simulink model "CF012A_GmStrtStop"  (R2013b)
settings: Solver=FixedStepDiscrete  SolverMode=SingleTasking  StartTime=0.0  StopTime=1  FixedStep=0.002  RelTol=1e-3
values from neighbouring files (symbols this model uses):
  CNV100MICROSECTOMILLISEC_MILLISECPERCNT_F32 = DataDict.Constant    [CF012A_GmStrtStop_DataDict.m]
  DISMOD_CNT_U08 = DataDict.Constant    [CF012A_GmStrtStop_DataDict.m]
  DISMODRATE_ULSPERSEC_F32 = DataDict.Constant    [CF012A_GmStrtStop_DataDict.m]
  FLTMOD_CNT_U08 = DataDict.Constant    [CF012A_GmStrtStop_DataDict.m]
  GmStrtStopEna = DataDict.Calibration    [CF012A_GmStrtStop_DataDict.m]
  GmStrtStopFltRateLim = DataDict.Calibration    [CF012A_GmStrtStop_DataDict.m]
  GmStrtStopMod1ToStopRateLim = DataDict.Calibration    [CF012A_GmStrtStop_DataDict.m]
  GmStrtStopNormRateLim = DataDict.Calibration    [CF012A_GmStrtStop_DataDict.m]
  GmStrtStopNormToMod1RateLim = DataDict.Calibration    [CF012A_GmStrtStop_DataDict.m]
  GmStrtStopStopAndMod2RateLim = DataDict.Calibration    [CF012A_GmStrtStop_DataDict.m]
  GmStrtStopStopMod1Tmr = DataDict.Calibration    [CF012A_GmStrtStop_DataDict.m]
  GmStrtStopStopMod2Tmr = DataDict.Calibration    [CF012A_GmStrtStop_DataDict.m]
  MOD1_CNT_U08 = DataDict.Constant    [CF012A_GmStrtStop_DataDict.m]
  MOD2_CNT_U08 = DataDict.Constant    [CF012A_GmStrtStop_DataDict.m]
  NORMMOD_CNT_U08 = DataDict.Constant    [CF012A_GmStrtStop_DataDict.m]
  STOPMOD_CNT_U08 = DataDict.Constant    [CF012A_GmStrtStop_DataDict.m]
  STRTSTOPRATEHILIM_ULSPERSEC_F32 = DataDict.Constant    [CF012A_GmStrtStop_DataDict.m]
  STRTSTOPRATELOWRLIM_ULSPERSEC_F32 = DataDict.Constant    [CF012A_GmStrtStop_DataDict.m]
  STRTSTOPSCAHILIM_ULS_F32 = DataDict.Constant    [CF012A_GmStrtStop_DataDict.m]
  STRTSTOPSCALOWRLIM_ULS_F32 = DataDict.Constant    [CF012A_GmStrtStop_DataDict.m]
undefined symbols (not defined in the file or in its folder): u2, u3, u4, u5
libraries: FixdToFloat x2, NxtrLim x2, simulink x2
(part 2 of 4)

== system CF012A_GmStrtStop/GmStrtStop/GmStrtStopPer1/DtrmnPrevActSt ==
  note: /*** Set PrevStrtStopSt read/write priority to fix bug, no software change required ***/
  StrtStopSt : Inport  RequirementInfo="{'linktype_rmi_doors' '0000c6e0 (/GM T1XX/SubSystem Specifications/Customer Functions/CF012 12V Start Stop)' '#186' 'true' 'REQ:  186' '' ; 'linktype_rmi_doors' '0000c6e0 (/GM T1XX/SubSystem Specifications/Customer Functions/CF012 12V Start Stop)' '#148' 'true' 'REQ:  148' '' ; 'linktype_rmi_doors' '0000c6e0 (/GM T1XX/SubSystem Specifications/Customer Functions/CF012 12V Start Stop)' '#148' 'true' 'REQ:  148' '' ; 'linktype_rmi_doors' '0000c6e0 (/GM T1XX/SubSystem Specifications/Customer Functions/CF012 12V Start Stop)' '#148' 'true' 'REQ:  148' '' ; 'linktype_rmi_doors' '0000c6e0 (/GM T1XX/SubSystem Specifications/Customer Functions/CF012 12V Start Stop)' '#148' 'true' 'REQ:  148' '' ; 'linktype_rmi_doors' '0000c6e0 (/GM T1XX/SubSystem Specifications/Customer Functions/CF012 12V Start Stop)' '#148' 'true' 'REQ:  148' '' ; 'linktype_rmi_doors' '0000c6e0 (/GM T1XX/SubSystem Specifications/Customer Functions/CF012 12V Start Stop)' '#148' 'true' 'REQ:  148' '' ; 'linktype_rmi_doors' '0000c6e0 (/GM T1XX/SubSystem Specifications/Customer Functions/CF012 12V Start Stop)' '#148' 'true' 'REQ:  148' '' } %GIDa_e4f48af0_6723_4855_972c_b2aebfcfadbe"
  CopyRight2 : Subsystem  Description=|  mask(Copyright Information){none=on}
      | Copyright info block.                                               
      |                                                                     
      | Place copyright information at the top of every subsystem in design.
      mask prompts: none "No parameters"
      mask help: Place copyright information at the top of every subsystem in design.
      mask Display:
      | NxtrConf = 'Nexteer Confidential';
      | 
      | sys = bdroot; %handle for the current model ("system")
      | first = get_param(sys,'Created');
      | if(isempty(first))
      |     first = datestr(now,'yyyy');
      | else
      |     first = first(end-3:end);  %year is last four digits
      | end
      | 
      | last = get_param(sys,'LastModifiedDate');
      | if isempty(last)
      |     last = datestr(now,'yyyy');
      | else
      |     last = last(end-3:end);
      | end
      | 
      | if strcmp(first,last)
      |     fprintf('%s -- Copyright %s Nexteer',NxtrConf,first)
      | else
      |     fprintf('%s -- %s%s- %s Nexteer',NxtrConf,char(169),first,last)
      | end
  Data Store Read : DataStoreRead  RequirementInfo="{'linktype_rmi_doors' '0000c6e0 (/GM T1XX/SubSystem Specifications/Customer Functions/CF012 12V Start Stop)' '#186' 'true' 'REQ:  186' '' ; 'linktype_rmi_doors' '0000c6e0 (/GM T1XX/SubSystem Specifications/Customer Functions/CF012 12V Start Stop)' '#148' 'true' 'REQ:  148' '' ; 'linktype_rmi_doors' '0000c6e0 (/GM T1XX/SubSystem Specifications/Customer Functions/CF012 12V Start Stop)' '#148' 'true' 'REQ:  148' '' ; 'linktype_rmi_doors' '0000c6e0 (/GM T1XX/SubSystem Specifications/Customer Functions/CF012 12V Start Stop)' '#148' 'true' 'REQ:  148' '' ; 'linktype_rmi_doors' '0000c6e0 (/GM T1XX/SubSystem Specifications/Customer Functions/CF012 12V Start Stop)' '#148' 'true' 'REQ:  148' '' ; 'linktype_rmi_doors' '0000c6e0 (/GM T1XX/SubSystem Specifications/Customer Functions/CF012 12V Start Stop)' '#148' 'true' 'REQ:  148' '' ; 'linktype_rmi_doors' '0000c6e0 (/GM T1XX/SubSystem Specifications/Customer Functions/CF012 12V Start Stop)' '#148' 'true' 'REQ:  148' '' ; 'linktype_rmi_doors' '0000c6e0 (/GM T1XX/SubSystem Specifications/Customer Functions/CF012 12V Start Stop)' '#148' 'true' 'REQ:  148' '' } %GIDa_4112967c_5abe_441b_ba9c_e70bf3192b6c"  Priority=0  DataStoreName=PrevStrtStopSt
      settings: AttributesFormatString=%<Priority>
  Data Store Write : DataStoreWrite  RequirementInfo="{'linktype_rmi_doors' '0000c6e0 (/GM T1XX/SubSystem Specifications/Customer Functions/CF012 12V Start Stop)' '#186' 'true' 'REQ:  186' '' ; 'linktype_rmi_doors' '0000c6e0 (/GM T1XX/SubSystem Specifications/Customer Functions/CF012 12V Start Stop)' '#148' 'true' 'REQ:  148' '' ; 'linktype_rmi_doors' '0000c6e0 (/GM T1XX/SubSystem Specifications/Customer Functions/CF012 12V Start Stop)' '#148' 'true' 'REQ:  148' '' ; 'linktype_rmi_doors' '0000c6e0 (/GM T1XX/SubSystem Specifications/Customer Functions/CF012 12V Start Stop)' '#148' 'true' 'REQ:  148' '' ; 'linktype_rmi_doors' '0000c6e0 (/GM T1XX/SubSystem Specifications/Customer Functions/CF012 12V Start Stop)' '#148' 'true' 'REQ:  148' '' ; 'linktype_rmi_doors' '0000c6e0 (/GM T1XX/SubSystem Specifications/Customer Functions/CF012 12V Start Stop)' '#148' 'true' 'REQ:  148' '' ; 'linktype_rmi_doors' '0000c6e0 (/GM T1XX/SubSystem Specifications/Customer Functions/CF012 12V Start Stop)' '#148' 'true' 'REQ:  148' '' ; 'linktype_rmi_doors' '0000c6e0 (/GM T1XX/SubSystem Specifications/Customer Functions/CF012 12V Start Stop)' '#148' 'true' 'REQ:  148' '' } %GIDa_cb98726f_60b3_46df_96ca_b94222df7bed"  Priority=1  DataStoreName=PrevStrtStopSt
      settings: AttributesFormatString=%<Priority>
  Data Store Write1 : DataStoreWrite  RequirementInfo="{'linktype_rmi_doors' '0000c6e0 (/GM T1XX/SubSystem Specifications/Customer Functions/CF012 12V Start Stop)' '#186' 'true' 'REQ:  186' '' ; 'linktype_rmi_doors' '0000c6e0 (/GM T1XX/SubSystem Specifications/Customer Functions/CF012 12V Start Stop)' '#148' 'true' 'REQ:  148' '' ; 'linktype_rmi_doors' '0000c6e0 (/GM T1XX/SubSystem Specifications/Customer Functions/CF012 12V Start Stop)' '#148' 'true' 'REQ:  148' '' ; 'linktype_rmi_doors' '0000c6e0 (/GM T1XX/SubSystem Specifications/Customer Functions/CF012 12V Start Stop)' '#148' 'true' 'REQ:  148' '' ; 'linktype_rmi_doors' '0000c6e0 (/GM T1XX/SubSystem Specifications/Customer Functions/CF012 12V Start Stop)' '#148' 'true' 'REQ:  148' '' ; 'linktype_rmi_doors' '0000c6e0 (/GM T1XX/SubSystem Specifications/Customer Functions/CF012 12V Start Stop)' '#148' 'true' 'REQ:  148' '' ; 'linktype_rmi_doors' '0000c6e0 (/GM T1XX/SubSystem Specifications/Customer Functions/CF012 12V Start Stop)' '#148' 'true' 'REQ:  148' '' ; 'linktype_rmi_doors' '0000c6e0 (/GM T1XX/SubSystem Specifications/Customer Functions/CF012 12V Start Stop)' '#148' 'true' 'REQ:  148' '' } %GIDa_3c095796_580b_4ffd_824f_51ea0e0332a4"  DataStoreName=PrevActSt
  Merge : Merge  RequirementInfo="{'linktype_rmi_doors' '0000c6e0 (/GM T1XX/SubSystem Specifications/Customer Functions/CF012 12V Start Stop)' '#186' 'true' 'REQ:  186' '' ; 'linktype_rmi_doors' '0000c6e0 (/GM T1XX/SubSystem Specifications/Customer Functions/CF012 12V Start Stop)' '#148' 'true' 'REQ:  148' '' ; 'linktype_rmi_doors' '0000c6e0 (/GM T1XX/SubSystem Specifications/Customer Functions/CF012 12V Start Stop)' '#148' 'true' 'REQ:  148' '' ; 'linktype_rmi_doors' '0000c6e0 (/GM T1XX/SubSystem Specifications/Customer Functions/CF012 12V Start Stop)' '#148' 'true' 'REQ:  148' '' ; 'linktype_rmi_doors' '0000c6e0 (/GM T1XX/SubSystem Specifications/Customer Functions/CF012 12V Start Stop)' '#148' 'true' 'REQ:  148' '' ; 'linktype_rmi_doors' '0000c6e0 (/GM T1XX/SubSystem Specifications/Customer Functions/CF012 12V Start Stop)' '#148' 'true' 'REQ:  148' '' ; 'linktype_rmi_doors' '0000c6e0 (/GM T1XX/SubSystem Specifications/Customer Functions/CF012 12V Start Stop)' '#148' 'true' 'REQ:  148' '' ; 'linktype_rmi_doors' '0000c6e0 (/GM T1XX/SubSystem Specifications/Customer Functions/CF012 12V Start Stop)' '#148' 'true' 'REQ:  148' '' } %GIDa_01ea55aa_64ba_4614_8fef_670c876545a6"
  PassLastSt : Subsystem  RequirementInfo="{'linktype_rmi_doors' '0000c6e0 (/GM T1XX/SubSystem Specifications/Customer Functions/CF012 12V Start Stop)' '#186' 'true' 'REQ:  186' '' ; 'linktype_rmi_doors' '0000c6e0 (/GM T1XX/SubSystem Specifications/Customer Functions/CF012 12V Start Stop)' '#148' 'true' 'REQ:  148' '' ; 'linktype_rmi_doors' '0000c6e0 (/GM T1XX/SubSystem Specifications/Customer Functions/CF012 12V Start Stop)' '#148' 'true' 'REQ:  148' '' ; 'linktype_rmi_doors' '0000c6e0 (/GM T1XX/SubSystem Specifications/Customer Functions/CF012 12V Start Stop)' '#148' 'true' 'REQ:  148' '' ; 'linktype_rmi_doors' '0000c6e0 (/GM T1XX/SubSystem Specifications/Customer Functions/CF012 12V Start Stop)' '#148' 'true' 'REQ:  148' '' ; 'linktype_rmi_doors' '0000c6e0 (/GM T1XX/SubSystem Specifications/Customer Functions/CF012 12V Start Stop)' '#148' 'true' 'REQ:  148' '' ; 'linktype_rmi_doors' '0000c6e0 (/GM T1XX/SubSystem Specifications/Customer Functions/CF012 12V Start Stop)' '#148' 'true' 'REQ:  148' '' ; 'linktype_rmi_doors' '0000c6e0 (/GM T1XX/SubSystem Specifications/Customer Functions/CF012 12V Start Stop)' '#148' 'true' 'REQ:  148' '' } %GIDa_88907860_9b17_4b86_96c1_9ce7d81e5492"  TreatAsAtomicUnit=on
  PassPrevLoopRes : Subsystem  RequirementInfo="{'linktype_rmi_doors' '0000c6e0 (/GM T1XX/SubSystem Specifications/Customer Functions/CF012 12V Start Stop)' '#186' 'true' 'REQ:  186' '' ; 'linktype_rmi_doors' '0000c6e0 (/GM T1XX/SubSystem Specifications/Customer Functions/CF012 12V Start Stop)' '#148' 'true' 'REQ:  148' '' ; 'linktype_rmi_doors' '0000c6e0 (/GM T1XX/SubSystem Specifications/Customer Functions/CF012 12V Start Stop)' '#148' 'true' 'REQ:  148' '' ; 'linktype_rmi_doors' '0000c6e0 (/GM T1XX/SubSystem Specifications/Customer Functions/CF012 12V Start Stop)' '#148' 'true' 'REQ:  148' '' ; 'linktype_rmi_doors' '0000c6e0 (/GM T1XX/SubSystem Specifications/Customer Functions/CF012 12V Start Stop)' '#148' 'true' 'REQ:  148' '' ; 'linktype_rmi_doors' '0000c6e0 (/GM T1XX/SubSystem Specifications/Customer Functions/CF012 12V Start Stop)' '#148' 'true' 'REQ:  148' '' ; 'linktype_rmi_doors' '0000c6e0 (/GM T1XX/SubSystem Specifications/Customer Functions/CF012 12V Start Stop)' '#148' 'true' 'REQ:  148' '' ; 'linktype_rmi_doors' '0000c6e0 (/GM T1XX/SubSystem Specifications/Customer Functions/CF012 12V Start Stop)' '#148' 'true' 'REQ:  148' '' } %GIDa_c43dcfaf_7e1c_468a_acca_d131cc0d12a7"  TreatAsAtomicUnit=on
  Relational Operator : RelationalOperator  RequirementInfo="{'linktype_rmi_doors' '0000c6e0 (/GM T1XX/SubSystem Specifications/Customer Functions/CF012 12V Start Stop)' '#186' 'true' 'REQ:  186' '' ; 'linktype_rmi_doors' '0000c6e0 (/GM T1XX/SubSystem Specifications/Customer Functions/CF012 12V Start Stop)' '#148' 'true' 'REQ:  148' '' ; 'linktype_rmi_doors' '0000c6e0 (/GM T1XX/SubSystem Specifications/Customer Functions/CF012 12V Start Stop)' '#148' 'true' 'REQ:  148' '' ; 'linktype_rmi_doors' '0000c6e0 (/GM T1XX/SubSystem Specifications/Customer Functions/CF012 12V Start Stop)' '#148' 'true' 'REQ:  148' '' ; 'linktype_rmi_doors' '0000c6e0 (/GM T1XX/SubSystem Specifications/Customer Functions/CF012 12V Start Stop)' '#148' 'true' 'REQ:  148' '' ; 'linktype_rmi_doors' '0000c6e0 (/GM T1XX/SubSystem Specifications/Customer Functions/CF012 12V Start Stop)' '#148' 'true' 'REQ:  148' '' ; 'linktype_rmi_doors' '0000c6e0 (/GM T1XX/SubSystem Specifications/Customer Functions/CF012 12V Start Stop)' '#148' 'true' 'REQ:  148' '' ; 'linktype_rmi_doors' '0000c6e0 (/GM T1XX/SubSystem Specifications/Customer Functions/CF012 12V Start Stop)' '#148' 'true' 'REQ:  148' '' } %GIDa_d7497edc_1bfd_4ac3_af9a_a8a8c06f0d57"  Operator=~=  OutDataTypeStr=boolean
  StrtStopSt_IF : If  RequirementInfo="{'linktype_rmi_doors' '0000c6e0 (/GM T1XX/SubSystem Specifications/Customer Functions/CF012 12V Start Stop)' '#186' 'true' 'REQ:  186' '' ; 'linktype_rmi_doors' '0000c6e0 (/GM T1XX/SubSystem Specifications/Customer Functions/CF012 12V Start Stop)' '#148' 'true' 'REQ:  148' '' ; 'linktype_rmi_doors' '0000c6e0 (/GM T1XX/SubSystem Specifications/Customer Functions/CF012 12V Start Stop)' '#148' 'true' 'REQ:  148' '' ; 'linktype_rmi_doors' '0000c6e0 (/GM T1XX/SubSystem Specifications/Customer Functions/CF012 12V Start Stop)' '#148' 'true' 'REQ:  148' '' ; 'linktype_rmi_doors' '0000c6e0 (/GM T1XX/SubSystem Specifications/Customer Functions/CF012 12V Start Stop)' '#148' 'true' 'REQ:  148' '' ; 'linktype_rmi_doors' '0000c6e0 (/GM T1XX/SubSystem Specifications/Customer Functions/CF012 12V Start Stop)' '#148' 'true' 'REQ:  148' '' ; 'linktype_rmi_doors' '0000c6e0 (/GM T1XX/SubSystem Specifications/Customer Functions/CF012 12V Start Stop)' '#148' 'true' 'REQ:  148' '' ; 'linktype_rmi_doors' '0000c6e0 (/GM T1XX/SubSystem Specifications/Customer Functions/CF012 12V Start Stop)' '#148' 'true' 'REQ:  148' '' } %GIDa_dbd55cf9_f195_4f11_95d6_87ed01c262a0"  IfExpression=u1
  PrevActSt : Outport  RequirementInfo="{'linktype_rmi_doors' '0000c6e0 (/GM T1XX/SubSystem Specifications/Customer Functions/CF012 12V Start Stop)' '#186' 'true' 'REQ:  186' '' ; 'linktype_rmi_doors' '0000c6e0 (/GM T1XX/SubSystem Specifications/Customer Functions/CF012 12V Start Stop)' '#148' 'true' 'REQ:  148' '' ; 'linktype_rmi_doors' '0000c6e0 (/GM T1XX/SubSystem Specifications/Customer Functions/CF012 12V Start Stop)' '#148' 'true' 'REQ:  148' '' ; 'linktype_rmi_doors' '0000c6e0 (/GM T1XX/SubSystem Specifications/Customer Functions/CF012 12V Start Stop)' '#148' 'true' 'REQ:  148' '' ; 'linktype_rmi_doors' '0000c6e0 (/GM T1XX/SubSystem Specifications/Customer Functions/CF012 12V Start Stop)' '#148' 'true' 'REQ:  148' '' ; 'linktype_rmi_doors' '0000c6e0 (/GM T1XX/SubSystem Specifications/Customer Functions/CF012 12V Start Stop)' '#148' 'true' 'REQ:  148' '' ; 'linktype_rmi_doors' '0000c6e0 (/GM T1XX/SubSystem Specifications/Customer Functions/CF012 12V Start Stop)' '#148' 'true' 'REQ:  148' '' ; 'linktype_rmi_doors' '0000c6e0 (/GM T1XX/SubSystem Specifications/Customer Functions/CF012 12V Start Stop)' '#148' 'true' 'REQ:  148' '' } %GIDa_a7fe661f_9dcc_4fc8_91f7_0b4e200f6a0d"
  wires:
  Relational Operator/1 -> StrtStopSt_IF/1
  Data Store Read/1 -> [PrevStrtStopSt], Relational Operator/2
  StrtStopSt_IF/1 -> PassPrevLoopRes/Action
  StrtStopSt_IF/2 -> PassLastSt/Action
  PassPrevLoopRes/1(PrevStrtStopSt) -> Merge/1
  PassLastSt/1(PrevActSt) -> Merge/2
  Merge/1 -> Data Store Write1/1, PrevActSt/1  "PrevActSt_Cnt_T_u08"
  [PrevStrtStopSt] -> PassPrevLoopRes/1(In)
  StrtStopSt/1 -> Data Store Write/1, Relational Operator/1

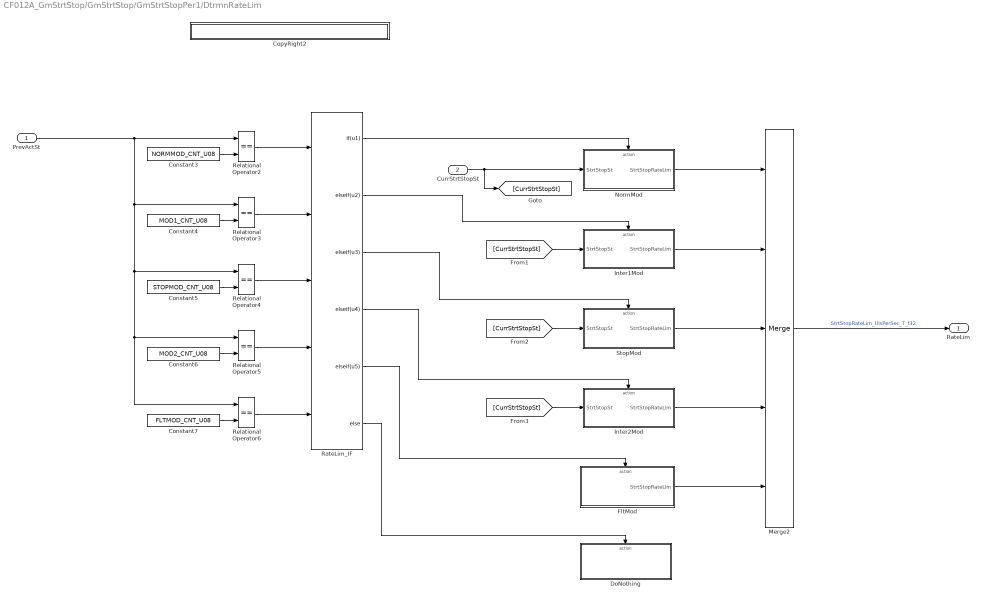
== system CF012A_GmStrtStop/GmStrtStop/GmStrtStopPer1/DtrmnRateLim ==
  PrevActSt : Inport
  CurrStrtStopSt : Inport  Port=2
  Constant3 : Constant  RequirementInfo="{'linktype_rmi_doors' '0000c6e0 (/GM T1XX/SubSystem Specifications/Customer Functions/CF012 12V Start Stop)' '#186' 'true' 'REQ:  186' '' ; 'linktype_rmi_doors' '0000c6e0 (/GM T1XX/SubSystem Specifications/Customer Functions/CF012 12V Start Stop)' '#196' 'true' 'REQ:  196' '' } %GIDa_269834e2_891d_44f8_bd1c_48fae9fdee15"  Value=NORMMOD_CNT_U08
  Constant4 : Constant  RequirementInfo="{'linktype_rmi_doors' '0000c6e0 (/GM T1XX/SubSystem Specifications/Customer Functions/CF012 12V Start Stop)' '#148' 'true' 'REQ:  148' '' ; 'linktype_rmi_doors' '0000c6e0 (/GM T1XX/SubSystem Specifications/Customer Functions/CF012 12V Start Stop)' '#188' 'true' 'REQ:  188' '' ; 'linktype_rmi_doors' '0000c6e0 (/GM T1XX/SubSystem Specifications/Customer Functions/CF012 12V Start Stop)' '#196' 'true' 'REQ:  196' '' } %GIDa_889a48a0_1b6c_471d_8a30_4fae277bcf4e"  Value=MOD1_CNT_U08
  Constant5 : Constant  RequirementInfo="{'linktype_rmi_doors' '0000c6e0 (/GM T1XX/SubSystem Specifications/Customer Functions/CF012 12V Start Stop)' '#190' 'true' 'REQ:  190' '' ; 'linktype_rmi_doors' '0000c6e0 (/GM T1XX/SubSystem Specifications/Customer Functions/CF012 12V Start Stop)' '#191' 'true' 'REQ:  191' '' ; 'linktype_rmi_doors' '0000c6e0 (/GM T1XX/SubSystem Specifications/Customer Functions/CF012 12V Start Stop)' '#196' 'true' 'REQ:  196' '' } %GIDa_4af1798e_c32a_476a_94ff_a04a59b8abca"  Value=STOPMOD_CNT_U08
  Constant6 : Constant  RequirementInfo="{'linktype_rmi_doors' '0000c6e0 (/GM T1XX/SubSystem Specifications/Customer Functions/CF012 12V Start Stop)' '#165' 'true' 'REQ:  165' '' ; 'linktype_rmi_doors' '0000c6e0 (/GM T1XX/SubSystem Specifications/Customer Functions/CF012 12V Start Stop)' '#196' 'true' 'REQ:  196' '' } %GIDa_fa3b7562_e0d9_484c_bab3_acc1dce49463"  Value=MOD2_CNT_U08
  Constant7 : Constant  RequirementInfo="{'linktype_rmi_doors' '0000c6e0 (/GM T1XX/SubSystem Specifications/Customer Functions/CF012 12V Start Stop)' '#196' 'true' 'REQ:  196' '' } %GIDa_11e42d8d_e247_4c4c_9f43_1e65bf7fd63c"  Value=FLTMOD_CNT_U08
  CopyRight2 : Subsystem  Description=|  mask(Copyright Information){none=on}
      | Copyright info block.                                               
      |                                                                     
      | Place copyright information at the top of every subsystem in design.
      mask prompts: none "No parameters"
      mask help: Place copyright information at the top of every subsystem in design.
      mask Display:
      | NxtrConf = 'Nexteer Confidential';
      | 
      | sys = bdroot; %handle for the current model ("system")
      | first = get_param(sys,'Created');
      | if(isempty(first))
      |     first = datestr(now,'yyyy');
      | else
      |     first = first(end-3:end);  %year is last four digits
      | end
      | 
      | last = get_param(sys,'LastModifiedDate');
      | if isempty(last)
      |     last = datestr(now,'yyyy');
      | else
      |     last = last(end-3:end);
      | end
      | 
      | if strcmp(first,last)
      |     fprintf('%s -- Copyright %s Nexteer',NxtrConf,first)
      | else
      |     fprintf('%s -- %s%s- %s Nexteer',NxtrConf,char(169),first,last)
      | end
  DoNothing : Subsystem  RequirementInfo={} %GIDa_ac4360b2_39ef_408f_bb15_008aee535945  TreatAsAtomicUnit=on
  FltMod : Subsystem
      settings: AttributesFormatString=Case 5. when PeviousState is FaultMode
  Inter1Mod : Subsystem  RequirementInfo="{'linktype_rmi_doors' '0000c6e0 (/GM T1XX/SubSystem Specifications/Customer Functions/CF012 12V Start Stop)' '#148' 'true' 'REQ:  148' '' ; 'linktype_rmi_doors' '0000c6e0 (/GM T1XX/SubSystem Specifications/Customer Functions/CF012 12V Start Stop)' '#188' 'true' 'REQ:  188' '' } %GIDa_aeeeecb0_b35b_4d36_9e8a_60c992b702c8"
      settings: AttributesFormatString=Case 2. when PreviousState is Intermediate1Mode
  Inter2Mod : Subsystem  RequirementInfo="{'linktype_rmi_doors' '0000c6e0 (/GM T1XX/SubSystem Specifications/Customer Functions/CF012 12V Start Stop)' '#165' 'true' 'REQ:  165' '' } %GIDa_17eeca2c_dc41_44f0_a34e_09f854028d20"
      settings: AttributesFormatString=Case 4. when PeviousState is Intermediate2Mode
  Merge2 : Merge  RequirementInfo="{'linktype_rmi_doors' '0000c6e0 (/GM T1XX/SubSystem Specifications/Customer Functions/CF012 12V Start Stop)' '#148' 'true' 'REQ:  148' '' } %GIDa_142071c0_28d8_458c_8f0d_290cc6845db0"  Inputs=5
  NormMod : Subsystem  RequirementInfo="{'linktype_rmi_doors' '0000c6e0 (/GM T1XX/SubSystem Specifications/Customer Functions/CF012 12V Start Stop)' '#186' 'true' 'REQ:  186' '' } %GIDa_4749cab3_b603_447e_b1c9_c0670dd4b4c5"
      settings: AttributesFormatString=Case 1. when PreviousState is NormalMode
  RateLim_IF : If  RequirementInfo="{'linktype_rmi_doors' '0000c6e0 (/GM T1XX/SubSystem Specifications/Customer Functions/CF012 12V Start Stop)' '#186' 'true' 'REQ:  186' '' ; 'linktype_rmi_doors' '0000c6e0 (/GM T1XX/SubSystem Specifications/Customer Functions/CF012 12V Start Stop)' '#148' 'true' 'REQ:  148' '' ; 'linktype_rmi_doors' '0000c6e0 (/GM T1XX/SubSystem Specifications/Customer Functions/CF012 12V Start Stop)' '#188' 'true' 'REQ:  188' '' ; 'linktype_rmi_doors' '0000c6e0 (/GM T1XX/SubSystem Specifications/Customer Functions/CF012 12V Start Stop)' '#190' 'true' 'REQ:  190' '' ; 'linktype_rmi_doors' '0000c6e0 (/GM T1XX/SubSystem Specifications/Customer Functions/CF012 12V Start Stop)' '#191' 'true' 'REQ:  191' '' ; 'linktype_rmi_doors' '0000c6e0 (/GM T1XX/SubSystem Specifications/Customer Functions/CF012 12V Start Stop)' '#165' 'true' 'REQ:  165' '' ; 'linktype_rmi_doors' '0000c6e0 (/GM T1XX/SubSystem Specifications/Customer Functions/CF012 12V Start Stop)' '#196' 'true' 'REQ:  196' '' } %GIDa_6dbd26ec_4dc9_4d09_b97e_31eb53c9da5c"  NumInputs=5  IfExpression=u1  ElseIfExpressions=u2,u3,u4,u5
  Relational Operator2 : RelationalOperator  RequirementInfo="{'linktype_rmi_doors' '0000c6e0 (/GM T1XX/SubSystem Specifications/Customer Functions/CF012 12V Start Stop)' '#186' 'true' 'REQ:  186' '' ; 'linktype_rmi_doors' '0000c6e0 (/GM T1XX/SubSystem Specifications/Customer Functions/CF012 12V Start Stop)' '#196' 'true' 'REQ:  196' '' } %GIDa_bc9dff2a_3ec8_47f3_b00b_e62fca045422"  Operator===  OutDataTypeStr=boolean
  Relational Operator3 : RelationalOperator  RequirementInfo="{'linktype_rmi_doors' '0000c6e0 (/GM T1XX/SubSystem Specifications/Customer Functions/CF012 12V Start Stop)' '#148' 'true' 'REQ:  148' '' ; 'linktype_rmi_doors' '0000c6e0 (/GM T1XX/SubSystem Specifications/Customer Functions/CF012 12V Start Stop)' '#188' 'true' 'REQ:  188' '' ; 'linktype_rmi_doors' '0000c6e0 (/GM T1XX/SubSystem Specifications/Customer Functions/CF012 12V Start Stop)' '#196' 'true' 'REQ:  196' '' } %GIDa_30044c4e_6525_47e0_90e3_b8ea8c4adf5f"  Operator===  OutDataTypeStr=boolean
  Relational Operator4 : RelationalOperator  RequirementInfo="{'linktype_rmi_doors' '0000c6e0 (/GM T1XX/SubSystem Specifications/Customer Functions/CF012 12V Start Stop)' '#190' 'true' 'REQ:  190' '' ; 'linktype_rmi_doors' '0000c6e0 (/GM T1XX/SubSystem Specifications/Customer Functions/CF012 12V Start Stop)' '#191' 'true' 'REQ:  191' '' ; 'linktype_rmi_doors' '0000c6e0 (/GM T1XX/SubSystem Specifications/Customer Functions/CF012 12V Start Stop)' '#196' 'true' 'REQ:  196' '' } %GIDa_bee7d651_229b_4e8e_a564_c9decdb49e6d"  Operator===  OutDataTypeStr=boolean
  Relational Operator5 : RelationalOperator  RequirementInfo="{'linktype_rmi_doors' '0000c6e0 (/GM T1XX/SubSystem Specifications/Customer Functions/CF012 12V Start Stop)' '#165' 'true' 'REQ:  165' '' ; 'linktype_rmi_doors' '0000c6e0 (/GM T1XX/SubSystem Specifications/Customer Functions/CF012 12V Start Stop)' '#196' 'true' 'REQ:  196' '' } %GIDa_742ca0cc_fdaf_42b6_ba60_c471effdb860"  Operator===  OutDataTypeStr=boolean
  Relational Operator6 : RelationalOperator  RequirementInfo="{'linktype_rmi_doors' '0000c6e0 (/GM T1XX/SubSystem Specifications/Customer Functions/CF012 12V Start Stop)' '#196' 'true' 'REQ:  196' '' } %GIDa_1350996a_bd33_449d_8727_2ff30dcaa48c"  Operator===  OutDataTypeStr=boolean
  StopMod : Subsystem  RequirementInfo="{'linktype_rmi_doors' '0000c6e0 (/GM T1XX/SubSystem Specifications/Customer Functions/CF012 12V Start Stop)' '#190' 'true' 'REQ:  190' '' ; 'linktype_rmi_doors' '0000c6e0 (/GM T1XX/SubSystem Specifications/Customer Functions/CF012 12V Start Stop)' '#191' 'true' 'REQ:  191' '' } %GIDa_99c1f662_a895_4901_a065_8cb300f6bb44"
      settings: AttributesFormatString=Case 3. when PeviousState is StopMode
  RateLim : Outport  RequirementInfo="{'linktype_rmi_doors' '0000c6e0 (/GM T1XX/SubSystem Specifications/Customer Functions/CF012 12V Start Stop)' '#148' 'true' 'REQ:  148' '' } %GIDa_e14362cd_9243_45cb_ba24_8c8b9f6b0966"
  wires:
  PrevActSt/1 -> Relational Operator6/1, Relational Operator5/1, Relational Operator4/1, Relational Operator3/1, Relational Operator2/1
  Constant3/1 -> Relational Operator2/2
  Constant4/1 -> Relational Operator3/2
  Constant5/1 -> Relational Operator4/2
  Constant6/1 -> Relational Operator5/2
  Constant7/1 -> Relational Operator6/2
  CurrStrtStopSt/1 -> [CurrStrtStopSt], NormMod/1(StrtStopSt)
  [CurrStrtStopSt] -> Inter2Mod/1(StrtStopSt)
  [CurrStrtStopSt] -> StopMod/1(StrtStopSt)
  [CurrStrtStopSt] -> Inter1Mod/1(StrtStopSt)
  FltMod/1(StrtStopRateLim) -> Merge2/5
  Inter2Mod/1(StrtStopRateLim) -> Merge2/4
  StopMod/1(StrtStopRateLim) -> Merge2/3
  Inter1Mod/1(StrtStopRateLim) -> Merge2/2
  NormMod/1(StrtStopRateLim) -> Merge2/1
  Relational Operator2/1 -> RateLim_IF/1
  Relational Operator3/1 -> RateLim_IF/2
  Relational Operator4/1 -> RateLim_IF/3
  Relational Operator5/1 -> RateLim_IF/4
  Relational Operator6/1 -> RateLim_IF/5
  RateLim_IF/1 -> NormMod/Action
  RateLim_IF/2 -> Inter1Mod/Action
  RateLim_IF/3 -> StopMod/Action
  RateLim_IF/4 -> Inter2Mod/Action
  RateLim_IF/5 -> FltMod/Action
  RateLim_IF/6 -> DoNothing/Action
  Merge2/1 -> RateLim/1  "StrtStopRateLim_UlsPerSec_T_f32"

== system CF012A_GmStrtStop/GmStrtStop/GmStrtStopPer1/Inter1ToStopModFlg ==
  Mod1 : Inport  RequirementInfo="{'linktype_rmi_doors' '0000c6e0 (/GM T1XX/SubSystem Specifications/Customer Functions/CF012 12V Start Stop)' '#149' 'true' 'REQ:  149' '' } %GIDa_416d315f_f051_4465_8213_88619b979863"
  CopyRight2 : Subsystem  Description=|  mask(Copyright Information){none=on}
      | Copyright info block.                                               
      |                                                                     
      | Place copyright information at the top of every subsystem in design.
      mask prompts: none "No parameters"
      mask help: Place copyright information at the top of every subsystem in design.
      mask Display:
      | NxtrConf = 'Nexteer Confidential';
      | 
      | sys = bdroot; %handle for the current model ("system")
      | first = get_param(sys,'Created');
      | first = first(end-3:end);  %year is last four digits
      | 
      | last = get_param(sys,'LastModifiedDate');
      | if isempty(last)
      |     last = datestr(now,'yyyy');
      | else
      |     last = last(end-3:end);
      | end
      | 
      | if strcmp(first,last)
      |     fprintf('%s -- Copyright %s Nexteer',NxtrConf,first)
      | else
      |     fprintf('%s -- %s%s- %s Nexteer',NxtrConf,char(169),first,last)
      | end
  Merge3 : Merge  RequirementInfo="{'linktype_rmi_doors' '0000c6e0 (/GM T1XX/SubSystem Specifications/Customer Functions/CF012 12V Start Stop)' '#149' 'true' 'REQ:  149' '' } %GIDa_54f564d7_cc60_4ede_bb38_14b0875fe6de"
  Mod1_IF : If  RequirementInfo="{'linktype_rmi_doors' '0000c6e0 (/GM T1XX/SubSystem Specifications/Customer Functions/CF012 12V Start Stop)' '#149' 'true' 'REQ:  149' '' } %GIDa_3dd33b8b_0b99_453d_ae2d_86699873d4a2"  IfExpression=u1
  RefTi : Subsystem  RequirementInfo="{'linktype_rmi_doors' '0000c6e0 (/GM T1XX/SubSystem Specifications/Customer Functions/CF012 12V Start Stop)' '#149' 'true' 'REQ:  149' '' } %GIDa_038d542a_5af1_408f_a6fe_c161387b2dbb"
  SpanTi : Subsystem  RequirementInfo="{'linktype_rmi_doors' '0000c6e0 (/GM T1XX/SubSystem Specifications/Customer Functions/CF012 12V Start Stop)' '#149' 'true' 'REQ:  149' '' } %GIDa_1641457f_302d_47f4_b79e_d0aab626086f"
  TranInter1ToStopMod : Outport  RequirementInfo="{'linktype_rmi_doors' '0000c6e0 (/GM T1XX/SubSystem Specifications/Customer Functions/CF012 12V Start Stop)' '#149' 'true' 'REQ:  149' '' } %GIDa_93df859a_5bad_41f5_b913_4124c0d822e2"
  wires:
  Mod1/1 -> Mod1_IF/1
  Mod1_IF/1 -> SpanTi/Action
  Mod1_IF/2 -> RefTi/Action
  SpanTi/1(TmrElpsdThd) -> Merge3/1
  RefTi/1(TmrElpsdThd) -> Merge3/2
  Merge3/1 -> TranInter1ToStopMod/1  "TranInter1ToStopMod_Cnt_T_logl"

== system CF012A_GmStrtStop/GmStrtStop/GmStrtStopPer1/Inter2ToStopModFlg ==
  Mod2 : Inport  RequirementInfo="{'linktype_rmi_doors' '0000c6e0 (/GM T1XX/SubSystem Specifications/Customer Functions/CF012 12V Start Stop)' '#156' 'true' 'REQ:  156' '' } %GIDa_2d46cf5e_b6dc_48ef_95b8_bbefab6693eb"
  CopyRight2 : Subsystem  Description=|  mask(Copyright Information){none=on}
      | Copyright info block.                                               
      |                                                                     
      | Place copyright information at the top of every subsystem in design.
      mask prompts: none "No parameters"
      mask help: Place copyright information at the top of every subsystem in design.
      mask Display:
      | NxtrConf = 'Nexteer Confidential';
      | 
      | sys = bdroot; %handle for the current model ("system")
      | first = get_param(sys,'Created');
      | first = first(end-3:end);  %year is last four digits
      | 
      | last = get_param(sys,'LastModifiedDate');
      | if isempty(last)
      |     last = datestr(now,'yyyy');
      | else
      |     last = last(end-3:end);
      | end
      | 
      | if strcmp(first,last)
      |     fprintf('%s -- Copyright %s Nexteer',NxtrConf,first)
      | else
      |     fprintf('%s -- %s%s- %s Nexteer',NxtrConf,char(169),first,last)
      | end
  Merge3 : Merge  RequirementInfo="{'linktype_rmi_doors' '0000c6e0 (/GM T1XX/SubSystem Specifications/Customer Functions/CF012 12V Start Stop)' '#156' 'true' 'REQ:  156' '' } %GIDa_de6abdd3_66c0_41fe_8abb_ae619c8e0af4"
  Mod2_IF : If  RequirementInfo="{'linktype_rmi_doors' '0000c6e0 (/GM T1XX/SubSystem Specifications/Customer Functions/CF012 12V Start Stop)' '#156' 'true' 'REQ:  156' '' } %GIDa_006b675f_7624_460b_82df_f7d2dd707aba"  IfExpression=u1
  RefTi : Subsystem  RequirementInfo="{'linktype_rmi_doors' '0000c6e0 (/GM T1XX/SubSystem Specifications/Customer Functions/CF012 12V Start Stop)' '#156' 'true' 'REQ:  156' '' } %GIDa_dfc3a3ca_de8b_45e9_b148_313862c3c7f8"
  SpanTi : Subsystem  RequirementInfo="{'linktype_rmi_doors' '0000c6e0 (/GM T1XX/SubSystem Specifications/Customer Functions/CF012 12V Start Stop)' '#156' 'true' 'REQ:  156' '' } %GIDa_c9a3910c_85c6_449f_bb80_c885fe95d931"
  TranInter2ToStopMod : Outport  RequirementInfo="{'linktype_rmi_doors' '0000c6e0 (/GM T1XX/SubSystem Specifications/Customer Functions/CF012 12V Start Stop)' '#156' 'true' 'REQ:  156' '' } %GIDa_15531fb1_0d3e_4b31_8dc3_211c42d6e663"
  wires:
  Merge3/1 -> TranInter2ToStopMod/1  "TranInter2ToStopMod_Cnt_T_logl"
  RefTi/1(TmrElpsdThd) -> Merge3/2
  SpanTi/1(TmrElpsdThd) -> Merge3/1
  Mod2_IF/2 -> RefTi/Action
  Mod2_IF/1 -> SpanTi/Action
  Mod2/1 -> Mod2_IF/1

== system CF012A_GmStrtStop/GmStrtStop/GmStrtStopPer1/PassDtrmnRateRes ==
  In : Inport
  Action Port : ActionPort  ActionType=else
  CopyRight2 : Subsystem  Description=|  mask(Copyright Information){none=on}
      | Copyright info block.                                               
      |                                                                     
      | Place copyright information at the top of every subsystem in design.
      mask prompts: none "No parameters"
      mask help: Place copyright information at the top of every subsystem in design.
      mask Display:
      | NxtrConf = 'Nexteer Confidential';
      | 
      | sys = bdroot; %handle for the current model ("system")
      | first = get_param(sys,'Created');
      | if(isempty(first))
      |     first = datestr(now,'yyyy');
      | else
      |     first = first(end-3:end);  %year is last four digits
      | end
      | 
      | last = get_param(sys,'LastModifiedDate');
      | if isempty(last)
      |     last = datestr(now,'yyyy');
      | else
      |     last = last(end-3:end);
      | end
      | 
      | if strcmp(first,last)
      |     fprintf('%s -- Copyright %s Nexteer',NxtrConf,first)
      | else
      |     fprintf('%s -- %s%s- %s Nexteer',NxtrConf,char(169),first,last)
      | end
  StrtStopRateLim : Outport
  wires:
  In/1 -> StrtStopRateLim/1

== system CF012A_GmStrtStop/GmStrtStop/GmStrtStopInit1/GetRefTmr100MicroSec32bit/CopyRight2 ==

== system CF012A_GmStrtStop/GmStrtStop/GmStrtStopPer1/DIModRate/CopyRight2 ==

== system CF012A_GmStrtStop/GmStrtStop/GmStrtStopPer1/DtrmnPrevActSt/CopyRight2 ==

== system CF012A_GmStrtStop/GmStrtStop/GmStrtStopPer1/DtrmnPrevActSt/PassLastSt ==
  Action Port : ActionPort  ActionType=else
  CopyRight2 : Subsystem  Description=|  mask(Copyright Information){none=on}
      | Copyright info block.                                               
      |                                                                     
      | Place copyright information at the top of every subsystem in design.
      mask prompts: none "No parameters"
      mask help: Place copyright information at the top of every subsystem in design.
      mask Display:
      | NxtrConf = 'Nexteer Confidential';
      | 
      | sys = bdroot; %handle for the current model ("system")
      | first = get_param(sys,'Created');
      | if(isempty(first))
      |     first = datestr(now,'yyyy');
      | else
      |     first = first(end-3:end);  %year is last four digits
      | end
      | 
      | last = get_param(sys,'LastModifiedDate');
      | if isempty(last)
      |     last = datestr(now,'yyyy');
      | else
      |     last = last(end-3:end);
      | end
      | 
      | if strcmp(first,last)
      |     fprintf('%s -- Copyright %s Nexteer',NxtrConf,first)
      | else
      |     fprintf('%s -- %s%s- %s Nexteer',NxtrConf,char(169),first,last)
      | end
  Data Store Read1 : DataStoreRead  DataStoreName=PrevActSt
  PrevActSt : Outport
  wires:
  Data Store Read1/1 -> PrevActSt/1

== system CF012A_GmStrtStop/GmStrtStop/GmStrtStopPer1/DtrmnPrevActSt/PassPrevLoopRes ==
  In : Inport
  Action Port : ActionPort  ActionType=then
  CopyRight2 : Subsystem  Description=|  mask(Copyright Information){none=on}
      | Copyright info block.                                               
      |                                                                     
      | Place copyright information at the top of every subsystem in design.
      mask prompts: none "No parameters"
      mask help: Place copyright information at the top of every subsystem in design.
      mask Display:
      | NxtrConf = 'Nexteer Confidential';
      | 
      | sys = bdroot; %handle for the current model ("system")
      | first = get_param(sys,'Created');
      | if(isempty(first))
      |     first = datestr(now,'yyyy');
      | else
      |     first = first(end-3:end);  %year is last four digits
      | end
      | 
      | last = get_param(sys,'LastModifiedDate');
      | if isempty(last)
      |     last = datestr(now,'yyyy');
      | else
      |     last = last(end-3:end);
      | end
      | 
      | if strcmp(first,last)
      |     fprintf('%s -- Copyright %s Nexteer',NxtrConf,first)
      | else
      |     fprintf('%s -- %s%s- %s Nexteer',NxtrConf,char(169),first,last)
      | end
  PrevStrtStopSt : Outport
  wires:
  In/1 -> PrevStrtStopSt/1

== system CF012A_GmStrtStop/GmStrtStop/GmStrtStopPer1/DtrmnRateLim/CopyRight2 ==

== system CF012A_GmStrtStop/GmStrtStop/GmStrtStopPer1/DtrmnRateLim/DoNothing ==
  note: /*** DoNothing ***/
  Action Port : ActionPort  ActionType=else
  CopyRight2 : Subsystem  Description=|  mask(Copyright Information){none=on}
      | Copyright info block.                                               
      |                                                                     
      | Place copyright information at the top of every subsystem in design.
      mask prompts: none "No parameters"
      mask help: Place copyright information at the top of every subsystem in design.
      mask Display:
      | NxtrConf = 'Nexteer Confidential';
      | 
      | sys = bdroot; %handle for the current model ("system")
      | first = get_param(sys,'Created');
      | if(isempty(first))
      |     first = datestr(now,'yyyy');
      | else
      |     first = first(end-3:end);  %year is last four digits
      | end
      | 
      | last = get_param(sys,'LastModifiedDate');
      | if isempty(last)
      |     last = datestr(now,'yyyy');
      | else
      |     last = last(end-3:end);
      | end
      | 
      | if strcmp(first,last)
      |     fprintf('%s -- Copyright %s Nexteer',NxtrConf,first)
      | else
      |     fprintf('%s -- %s%s- %s Nexteer',NxtrConf,char(169),first,last)
      | end

== system CF012A_GmStrtStop/GmStrtStop/GmStrtStopPer1/DtrmnRateLim/FltMod ==
  note: Transfer from FaultMode to NormalMode
  Action Port : ActionPort  ActionType=elseif
  Constant2 : Constant  RequirementInfo="{'linktype_rmi_doors' '0000c6e0 (/GM T1XX/SubSystem Specifications/Customer Functions/CF012 12V Start Stop)' '#196' 'true' 'REQ:  196' '' } %GIDa_b2615cf3_94f6_4d1f_b898_3ca59cf06a7b"  Value=GmStrtStopNormRateLim  OutDataTypeStr=single
  CopyRight2 : Subsystem  Description=|  mask(Copyright Information){none=on}
      | Copyright info block.                                               
      |                                                                     
      | Place copyright information at the top of every subsystem in design.
      mask prompts: none "No parameters"
      mask help: Place copyright information at the top of every subsystem in design.
      mask Display:
      | NxtrConf = 'Nexteer Confidential';
      | 
      | sys = bdroot; %handle for the current model ("system")
      | first = get_param(sys,'Created');
      | if(isempty(first))
      |     first = datestr(now,'yyyy');
      | else
      |     first = first(end-3:end);  %year is last four digits
      | end
      | 
      | last = get_param(sys,'LastModifiedDate');
      | if isempty(last)
      |     last = datestr(now,'yyyy');
      | else
      |     last = last(end-3:end);
      | end
      | 
      | if strcmp(first,last)
      |     fprintf('%s -- Copyright %s Nexteer',NxtrConf,first)
      | else
      |     fprintf('%s -- %s%s- %s Nexteer',NxtrConf,char(169),first,last)
      | end
  StrtStopRateLim : Outport  RequirementInfo="{'linktype_rmi_doors' '0000c6e0 (/GM T1XX/SubSystem Specifications/Customer Functions/CF012 12V Start Stop)' '#196' 'true' 'REQ:  196' '' } %GIDa_c78b1048_220b_4bb1_b28c_596ee263050b"
  wires:
  Constant2/1 -> StrtStopRateLim/1
